simulink library "INT_ActMod_TrqCalc"  (R2016b)
settings: Solver=VariableStepAuto  StartTime=0.0  StopTime=10.0  RelTol=1e-3
settings Model: Creator=zhoutinglin  LastModifiedBy=zhoutinglin

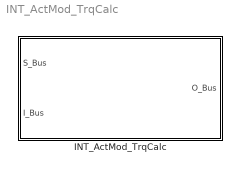
== system INT_ActMod_TrqCalc ==
  INT_ActMod_TrqCalc : Subsystem

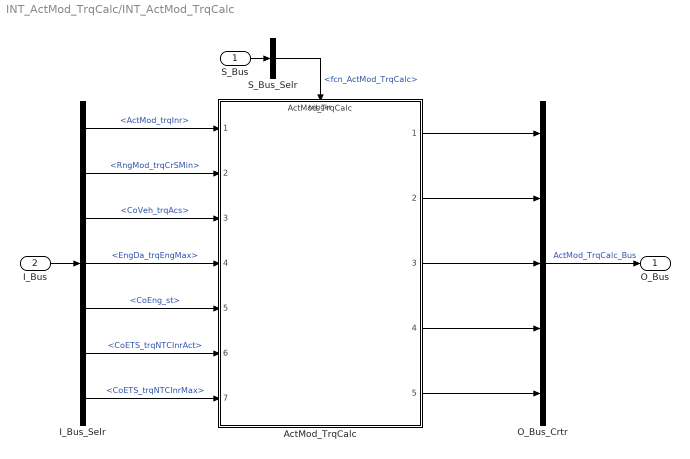
== system INT_ActMod_TrqCalc/INT_ActMod_TrqCalc ==
  S_Bus : Inport
  I_Bus : Inport  Port=2
  ActMod_TrqCalc : ModelReference  ModelNameDialog=ActMod_TrqCalc  SimulationMode=Normal  ModelReferenceVersion=1.11  TriggerPortName=function  TriggerPortTriggerType=function-call  TriggerPortStatesWhenEnabling=held
  I_Bus_Selr : BusSelector  OutputSignals=ActMod_trqInr,RngMod_trqCrSMin,CoVeh_trqAcs,EngDa_trqEngMax,CoEng_st,CoETS_trqNTCInrAct,CoETS_trqNTCInrMax
  O_Bus_Crtr : BusCreator  Inputs=5
  S_Bus_Selr : BusSelector  OutputSignals=fcn_ActMod_TrqCalc
  O_Bus : Outport
  wires:
  S_Bus_Selr/1 -> ActMod_TrqCalc/Trigger  "<fcn_ActMod_TrqCalc>"
  S_Bus/1 -> S_Bus_Selr/1
  I_Bus/1 -> I_Bus_Selr/1
  I_Bus_Selr/1 -> ActMod_TrqCalc/1  "<ActMod_trqInr>"
  I_Bus_Selr/2 -> ActMod_TrqCalc/2  "<RngMod_trqCrSMin>"
  I_Bus_Selr/3 -> ActMod_TrqCalc/3  "<CoVeh_trqAcs>"
  I_Bus_Selr/4 -> ActMod_TrqCalc/4  "<EngDa_trqEngMax>"
  I_Bus_Selr/5 -> ActMod_TrqCalc/5  "<CoEng_st>"
  I_Bus_Selr/6 -> ActMod_TrqCalc/6  "<CoETS_trqNTCInrAct>"
  I_Bus_Selr/7 -> ActMod_TrqCalc/7  "<CoETS_trqNTCInrMax>"
  O_Bus_Crtr/1 -> O_Bus/1  "ActMod_TrqCalc_Bus"
  ActMod_TrqCalc/1 -> O_Bus_Crtr/1
  ActMod_TrqCalc/2 -> O_Bus_Crtr/2
  ActMod_TrqCalc/3 -> O_Bus_Crtr/3
  ActMod_TrqCalc/4 -> O_Bus_Crtr/4
  ActMod_TrqCalc/5 -> O_Bus_Crtr/5
